simulink model "example"  (R2018b)
settings: Solver=VariableStepAuto  StartTime=0.0  StopTime=10.0  RelTol=1e-3
settings Model: Creator=wangh  LastModifiedBy=wangh

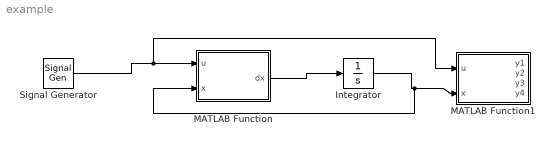
== system example ==
  Integrator : Integrator
  MATLAB Function : MATLAB Function  TreatAsAtomicUnit=on
  MATLAB Function1 : MATLAB Function  TreatAsAtomicUnit=on
  Signal Generator : SignalGenerator  Units=rad/sec
  wires:
  Signal Generator/1 -> MATLAB Function1/1(u), MATLAB Function/1(u)
  MATLAB Function/1(dx) -> Integrator/1
  Integrator/1 -> MATLAB Function/2(x), MATLAB Function1/2(x)

== matlab function example/MATLAB Function1 ==
  data: u input; y1 output; x input; y2 output; y3 output; y4 output
function [y1, y2, y3, y4] = fcn(u,x)


end

== matlab function example/MATLAB Function ==
  data: u input; dx output; x input
function dx = fcn(u,x)


end
